simulink model "20240115_HVDCMMCInterconnection"  (R2023b)
settings: Solver=FixedStepDiscrete  StartTime=0.0  StopTime=2  FixedStep=Ts_Power  RelTol=1e-4  EnableMultiTasking=on
PreLoadFcn:
  | HVDCMMCInterconnectionParam
StartFcn:
  | tic
StopFcn:
  | toc
values from neighbouring files (symbols this model uses):
  C_PM = 1.758e-3    (= 0.001758)    [HVDCMMCInterconnectionParam.m]
  Cg = 50e-9    (= 5e-08)    [HVDCMMCInterconnectionParam.m]
  D_R = 0.001    [HVDCMMCInterconnectionParam.m]
  D_Rs = 1e8    (= 100000000)    [HVDCMMCInterconnectionParam.m]
  D_Vf = 0    [HVDCMMCInterconnectionParam.m]
  Fnom = 50    [HVDCMMCInterconnectionParam.m]
  HRM = 2    [HVDCMMCInterconnectionParam.m]
  Ki_Ireg = 6    [HVDCMMCInterconnectionParam.m]
  Ki_Preg = 1.0    (= 1)    [HVDCMMCInterconnectionParam.m]
  Ki_Qreg = 1.0    (= 1)    [HVDCMMCInterconnectionParam.m]
  Ki_VDCreg = 100    [HVDCMMCInterconnectionParam.m]
  Kp_Ireg = 0.6    [HVDCMMCInterconnectionParam.m]
  Kp_Preg = 0.5/3    (= 0.166666666667)    [HVDCMMCInterconnectionParam.m]
  Kp_Qreg = 0.5/3    (= 0.166666666667)    [HVDCMMCInterconnectionParam.m]
  Kp_VDCreg = 4    [HVDCMMCInterconnectionParam.m]
  L_cable = 15e-3    (= 0.015)    [HVDCMMCInterconnectionParam.m]
  Larm = Larm_pu*(Zb_ac/(2*pi*Fnom))    [HVDCMMCInterconnectionParam.m]
  Lff = Larm_pu/2    (= 0.075)    [HVDCMMCInterconnectionParam.m]
  Limits_Ireg = [ 2.0  -2.0]    [HVDCMMCInterconnectionParam.m]
  Limits_Preg = [ 1.2, 0.8 ]    [HVDCMMCInterconnectionParam.m]
  Limits_Qreg = [ 0.25, -0.25 ]    [HVDCMMCInterconnectionParam.m]
  Limits_VDCreg = [ 2.0  -2.0]    [HVDCMMCInterconnectionParam.m]
  Lxfo = 0.12    [HVDCMMCInterconnectionParam.m]
  Nb_PM = 36    [HVDCMMCInterconnectionParam.m]
  Pnom = 1000e6    (= 1000000000)    [HVDCMMCInterconnectionParam.m]
  R_cable = 0.5    [HVDCMMCInterconnectionParam.m]
  R_startup = 400    [HVDCMMCInterconnectionParam.m]
  Rarm = Rarm_pu*Zb_ac    [HVDCMMCInterconnectionParam.m]
  Rff = Rarm_pu/2    (= 0.00075)    [HVDCMMCInterconnectionParam.m]
  Rg = 100    [HVDCMMCInterconnectionParam.m]
  Rxfo = 0.003    [HVDCMMCInterconnectionParam.m]
  Slope_Pref = 0.5    [HVDCMMCInterconnectionParam.m]
  Slope_Qref = 0.5    [HVDCMMCInterconnectionParam.m]
  Slope_Vdc_ref = Vnom_dc/5    (= 128000)    [HVDCMMCInterconnectionParam.m]
  Tbrk1_On = 0.1    [HVDCMMCInterconnectionParam.m]
  Tbrk2_On = 1.0    (= 1)    [HVDCMMCInterconnectionParam.m]
  Tdeblock = 1.5    [HVDCMMCInterconnectionParam.m]
  Tfault = 9999    [HVDCMMCInterconnectionParam.m]
  Ton_Converter2 = 4    [HVDCMMCInterconnectionParam.m]
  Ton_PQreg = 4    [HVDCMMCInterconnectionParam.m]
  Ton_VDCreg = 1.5    [HVDCMMCInterconnectionParam.m]
  Ts = Ts_Control    (= 4e-05)    [HVDCMMCInterconnectionParam.m]
  Ts_Control = 40e-6    (= 4e-05)    [HVDCMMCInterconnectionParam.m]
  Ts_Power = 20e-6    (= 2e-05)    [HVDCMMCInterconnectionParam.m]
  Vb_ac = sqrt(2/3)*Vnom_sec    [HVDCMMCInterconnectionParam.m]
  Vb_dc = Vnom_dc    (= 640000)    [HVDCMMCInterconnectionParam.m]
  Vc0_PM = 0    [HVDCMMCInterconnectionParam.m]
  Vnom_dc = 640e3    (= 640000)    [HVDCMMCInterconnectionParam.m]
  Vnom_prim = 400e3    (= 400000)    [HVDCMMCInterconnectionParam.m]
  Vnom_sec = 333e3    (= 333000)    [HVDCMMCInterconnectionParam.m]
  w = 2*pi*Fnom    (= 314.159265359)    [HVDCMMCInterconnectionParam.m]
undefined symbols (not defined in the file or in its folder): ACDC3, DiscIntNeverNeededParam, gcbh, Pcc, sps_AC, sps_rtmsupport
libraries: simulink x38, spsControlledVoltageSourceLib x36, spsCurrentMeasurementLib x36, spsSeriesRLCBranchLib x26, spsDiodeLib x20, spsVoltageMeasurementLib x18, spsThreePhaseSeriesRLCBranchLib x7, spsGroundLib x7, spsHalfBridgeMMCmodel x4, powerlib_extras x3, spsMultimeterLib x3, spsThreePhaseBreakerLib x2
(part 1 of 7)
settings Model: Creator=The MathWorks, Inc.  LastModifiedBy=rober
settings SolverCC: ConcurrentTasks=on  ZeroCrossAlgorithm=Adaptive  InsertRTBMode=Always
settings DataIOCC: SaveFormat=StructureWithTime  SaveOutput=off  SignalLogging=off  DSMLogging=off  SaveTime=off  ReturnWorkspaceOutputs=off
settings OptimizationCC: ReuseModelBlockBuffer=off  ExpressionDepthLimit=2147483647  LifeSpan=inf
settings DebuggingCC: UnderspecifiedInitializationDetection=Classic  MergeDetectMultiDrivingBlocksExec=none  SolverPrmCheckMsg=warning  FcnCallInpInsideContextMsg=warning  AllowSymbolicDim=off  StateNameClashWarn=warning  SFUnexpectedBacktrackingDiag=warning  SFNoUnconditionalDefaultTransitionDiag=warning  SFExecutionAtInitializationDiag=none  ArithmeticOperatorsInVariantConditions=warning
settings HardwareCC: ProdBitPerPointer=32  ProdBitPerSizeT=32  ProdBitPerPtrDiffT=32  ProdLargestAtomicFloat=None  ProdIntDivRoundTo=Undefined  ProdEndianess=Unspecified  ProdWordSize=32  ProdHWDeviceType=32-bit Generic
settings ModelReferenceCC: EnableRefExpFcnMdlSchedulingChecks=on  EnableParallelModelReferenceBuilds=on  ModelReferenceMinAlgLoopOccurrences=on  PropagateSignalLabelsOutOfModel=off  UseModelRefSolver=on
settings SFSimCC: SimUseLocalCustomCode=off  CustomCodeUndefinedFunction=UseInterfaceOnly
settings RTWCC: RTWUseLocalCustomCode=off
settings CodeAppCC: StateflowObjectComments=on
settings GRTTargetCC: CombineOutputUpdateFcns=off  GRTInterface=on
settings ConfigComp: CovMetricSettings=dw  CovSaveCumulativeToWorkspaceVar=on  CovSaveSingleToWorkspaceVar=on  CovExternalEMLEnable=off
settings SimscapeCC: SimscapeNormalizeSystem=off

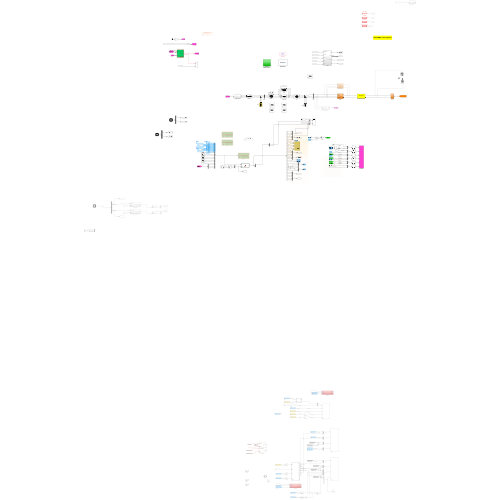
[thumbnail: Simulink's stored preview of the top-level diagram]
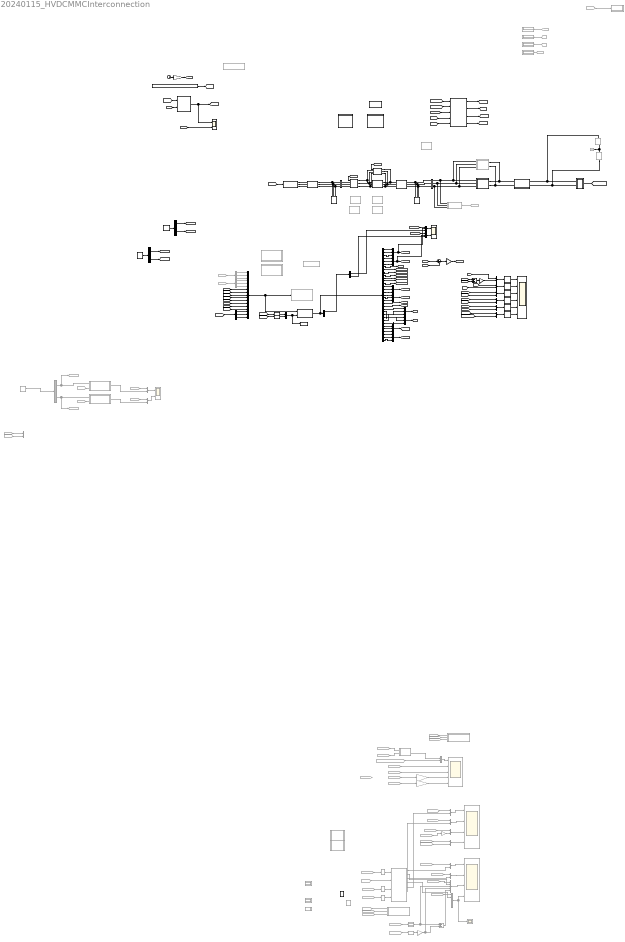
== system 20240115_HVDCMMCInterconnection ==
  note: HVDC-MMC Control System
  3ph SM1 : Subsystem  Commented=on
  3ph SM2 : Subsystem  Commented=on
  Add1 : Sum  Inputs=-+
  BRK_CTRL : Subsystem  Commented=on
  BRK_CTRL1 : Subsystem  Commented=on
  Brk1 : spsThreePhaseBreakerLib/Three-Phase Breaker  InitialState=open  SwitchA=on  SwitchB=on  SwitchC=on  SwitchTimes=0.1  External=on  BreakerResistance=0.01  SnubberResistance=1e6  SnubberCapacitance=inf  Measurements=Breaker voltages and currents
  Brk1_RS : spsThreePhaseSeriesRLCBranchLib/Three-Phase Series RLC Branch  Commented=on  LConnTagsString=A|B|C  RConnTagsString=A|B|C  BranchType=R  Resistance=1e6  Inductance=Vnom_prim^2 / Pcc / (2*pi*Fnom)  Capacitance=1e-6  Measurements=None
  Brk1_Ron : spsThreePhaseSeriesRLCBranchLib/Three-Phase Series RLC Branch  Commented=on  LConnTagsString=A|B|C  RConnTagsString=A|B|C  BranchType=R  Resistance=0.009  Inductance=Vnom_prim^2 / Pcc / (2*pi*Fnom)  Capacitance=1e-6  Measurements=None
  Brk2 : spsThreePhaseBreakerLib/Three-Phase Breaker  InitialState=open  SwitchA=on  SwitchB=on  SwitchC=on  SwitchTimes=[30/60]*10000  External=on  BreakerResistance=0.011  SnubberResistance=1e6  SnubberCapacitance=inf  Measurements=Breaker voltages and currents
  Brk2_RS : spsThreePhaseSeriesRLCBranchLib/Three-Phase Series RLC Branch  Commented=on  LConnTagsString=A|B|C  RConnTagsString=A|B|C  BranchType=R  Resistance=1e6  Inductance=Vnom_prim^2 / Pcc / (2*pi*Fnom)  Capacitance=1e-6  Measurements=None
  Brk2_Ron : spsThreePhaseSeriesRLCBranchLib/Three-Phase Series RLC Branch  Commented=on  LConnTagsString=A|B|C  RConnTagsString=A|B|C  BranchType=R  Resistance=0.011  Inductance=Vnom_prim^2 / Pcc / (2*pi*Fnom)  Capacitance=1e-6  Measurements=None
  COMPARE1 : Scope  NumInputPorts=6
  Cast To Double : DataTypeConversion  OutDataTypeStr=double  SaturateOnIntegerOverflow=off  RndMeth=Floor
  Cast To Double1 : DataTypeConversion  OutDataTypeStr=double  SaturateOnIntegerOverflow=off  RndMeth=Floor
  Clock : Clock
  Constant3 : Constant  Value=complex( [[ 0 Vnom_prim*sqrt(2/3); 0 0; 0 0] zeros(3,HRM-1) ])
  Control : Subsystem
  Conv 2 : Subsystem
      settings: PortSchema="{\"entries\":[{\"content\":{\"sides\":[{\"content\":{\"connectorIds\":[\"LConn1\",\"LConn2\"]},\"type\":\"ConnectorPlacement.EquallySpacedRectSide\",\"uuid\":\"34e68c3c-08e2-4036-96f4-bd6ca1a4adc7\"},{\"content\":{\"connectorIds\":[\"In1\"],\"side\":\"RIGHT\"},\"type\":\"ConnectorPlacement.EquallySpacedRectSide\",\"uuid\":\"8026f2da-b291-4e86-8efa-4dfa5391ad34\"},{\"content\":{\"side\":\"TOP\"},\"type\":\"ConnectorPlacement.EquallySpacedRectSide\",\"uuid\":\"2a5049d1-3deb-4ece-8237-adb3b31cd77f\"}]},\"type\":\"ConnectorPlacement.EquallySpacedConnector\",\"uuid\":\"95075630-e580-4539-9cf3-c9c75bab0a7f\"}],\"packageUris\":[\"http://schema.mathworks.com/mf0/Connector/R2020b\"],\"version\":\"1.0\"}"
  DC & converter 2 : Subsystem
      mask Display: disp('DC circuit')
  DQn->ABC : MATLAB Function  TreatAsAtomicUnit=on  SystemSampleTime=Ts_Power  mask{N=HRM}
      mask prompts: N "Harmonic order:"
  DSS : Subsystem  Commented=on  SystemSampleTime=Ts_Power  mask{A=ACDC3.A, B=ACDC3.B, C=ACDC3.C, D=ACDC3.D, InitVec=ACDC3.x0, dt=Ts_Power, DQSYM=off, N=HRM, Ws=w}
      mask prompts: InitVec "Initial condition:"; dt "Time step (s):"; N "Harmonic number:"; Ws "Angular frequency (1/rad):"
      mask init:
      | % I = eye(size(A,1));
      | % INVR = I/(I-A*dt/2);
      | % Ad1 = INVR*(I+A*dt/2);
      | % Bd1 = INVR*B*dt/2;
      | % Cd1 = C*Ad1;
      | % Dd11 = C*INVR*B*dt/2+D;
      | % Dd12 = C*INVR*B*dt/2;
      | 
      |     I = eye(size(A,1));
      |     INVR = I/(I-A*dt/2);
      |     Ad1 = INVR*(I+A*dt/2);
      |     Bd1 = INVR*B;
      |     Cd1 = C*INVR*dt;
      |     Dd1 = Cd1*B/2 + D;
      | 
      | DQSYM = get_param(gcb,'DQSYM');
      | 
      | comp = 0;
      | 
      | if(strcmp(DQSYM,'on'))
      | 
      | %Calculating the PNZ matrices
      | 
      |     a = -0.5+0.866i;
      |     a2 = -0.5-0.866i;
      |     Sas = [1,a,a2;1,a2,a;1,1,1]/3;
      | 
      |     arows = size(Ad1,1)/3; %signal size
      |     acols = size(Ad1,2)/3; %signal size
      | 
      |     brows = size(Bd1,1)/3; %signal size
      |     bcols = size(Bd1,2)/3; %signal size
      | 
      |     crows = size(Cd1,1)/3; %signal size
      |     ccols = size(Cd1,2)/3; %signal size
      | 
      |     d1rows = size(Dd1,1)/3; %signal size
      |     d1cols = size(Dd1,2)/3; %signal size
      | 
      |     %%%%%%%%%%%%%%%%%%%%%%% Check for inconsistencies  %%%%%%%%%%%%%%%%%%%%%%%
      | 
      |     szMatA = size(A,1);
      |     iL = eye(szMatA);
      |     szMatiL = size(iL,1);
      | 
      |     if(szMatiL ~= szMatA || size(A,1) ~= size(A,2) || size(iL,1) ~= size(iL,2))
      |         error('[Int_DQN_Mat/swFeedback] check matrix A size!');
      |     end
      | 
      |     if(arows ~= brows || acols ~= ccols || crows ~= d1rows || bcols ~= d1cols)
      |         error('[Int_DQN_Mat/Initialize] the sizes of the state-space matrices!');
      |     end
      | 
      |     %%%%%%%%%%%%%%%%%%%%%%%%%%%%%%%%%%%%%%%%%%%%%%%%%%%%%%%%%%%%%%%
      | 
      | 
      |     %%%%%%%%%%%%%%%%%%%%%%% A --> Bpnz %%%%%%%%%%%%%%%%%%%%%%%
      |     Adc = complex(zeros(3*arows,3*acols));
      | 
      |     for i = 1 : arows
      |         for j = 1 : acols
      |             Adc((1:3) + (i-1)*3,(1:3) + (j-1)*3) = Sas*Ad1((1:3) + (i-1)*3,(1:3) + (j-1)*3)/Sas;
      |             %Adc((1:3) + (i-1)*3,(1:3) + (j-1)*3) = diag(diag(real(Adc((1:3) + (i-1)*3,(1:3) + (j-1)*3))));
      |             %Adc((1:3) + (i-1)*3,(1:3) + (j-1)*3) = diag(diag((Adc((1:3) + (i-1)*3,(1:3) + (j-1)*3))));
      | 
      |         end
      |     end
      |     %%%%%%%%%%%%%%%%%%%%%%%%%%%%%%%%%%%%%%%%%%%%%%%%%%%%%%%%%%%%%%%
      | 
      |     %%%%%%%%%%%%%%%%%%%%%%% B --> Bpnz %%%%%%%%%%%%%%%%%%%%%%%
      | 
      |     Bdc = complex(zeros(3*brows,3*bcols));
      | 
      |     for i = 1 : brows
      |         for j = 1 : bcols
      |             Bdc((1:3) + (i-1)*3,(1:3) + (j-1)*3) = Sas*Bd1((1:3) + (i-1)*3,(1:3) + (j-1)*3)/Sas;
      |             %Bdc((1:3) + (i-1)*3,(1:3) + (j-1)*3) = diag(diag(real(Bdc((1:3) + (i-1)*3,(1:3) + (j-1)*3))));
      |             %Bdc((1:3) + (i-1)*3,(1:3) + (j-1)*3) = diag(diag((Bdc((1:3) + (i-1)*3,(1:3) + (j-1)*3))));
      | 
      |         end
      |     end
      |     %%%%%%%%%%%%%%%%%%%%%%%%%%%%%%%%%%%%%%%%%%%%%%%%%%%%%%%%%%%%%%%
      | 
      |     %%%%%%%%%%%%%%%%%%%%%%% C --> Cpnz %%%%%%%%%%%%%%%%%%%%%%%
      | 
      |     Cdc = complex(zeros(3*crows,3*ccols));
      | 
      |     for i = 1 : crows
      |         for j = 1 : ccols
      |             Cdc((1:3) + (i-1)*3,(1:3) + (j-1)*3) = Sas*Cd1((1:3) + (i-1)*3,(1:3) + (j-1)*3)/Sas;
      |             %Cdc((1:3) + (i-1)*3,(1:3) + (j-1)*3) = diag(diag(real(Cdc((1:3) + (i-1)*3,(1:3) + (j-1)*3))));
      |             %Cdc((1:3) + (i-1)*3,(1:3) + (j-1)*3) = diag(diag((Cdc((1:3) + (i-1)*3,(1:3) + (j-1)*3))));
      |         end
      |     end
      |     %%%%%%%%%%%%%%%%%%%%%%%%%%%%%%%%%%%%%%%%%%%%%%%%%%%%%%%%%%%%%%%
      | 
      |     
      |     %%%%%%%%%%%%%%%%%%%%%%% D1 --> Cpnz %%%%%%%%%%%%%%%%%%%%%%%
      | 
      |     Ddc = complex(zeros(3*d1rows,3*d1cols));
      | 
      |     for i = 1 : d1rows
      |         for j = 1 : d1cols
      |             Ddc((1:3) + (i-1)*3,(1:3) + (j-1)*3) = Sas*Dd1((1:3) + (i-1)*3,(1:3) + (j-1)*3)/Sas;
      |             %Ddc1((1:3) + (i-1)*3,(1:3) + (j-1)*3) = diag(diag(real(Ddc1((1:3) + (i-1)*3,(1:3) + (j-1)*3))));
      |             %Ddc((1:3) + (i-1)*3,(1:3) + (j-1)*3) = diag(diag((Ddc((1:3) + (i-1)*3,(1:3) + (j-1)*3))));
      |         end
      |     end
      |     %%%%%%%%%%%%%%%%%%%%%%%%%%%%%%%%%%%%%%%%%%%%%%%%%%%%%%%%%%%%%%%
      | 
      |     Adc(abs(Adc)<2*eps) = 0;
      |     Bdc(abs(Bdc)<2*eps) = 0;
      |     Cdc(abs(Cdc)<2*eps) = 0;
      |     Ddc(abs(Ddc)<2*eps) = 0;
      | 
      |     InitVec_c = complex(zeros(brows*3,N+1));
      | 
      | 
      |     if(~isempty(InitVec))
      |         if(mod(numel(InitVec),3)~=0) 
      |             warning('[SS_DQNc_Mat] InitVec with wrong size --> needs to be a multiple of 3!'); 
      | 
      |         else
      |             for k = 1 : numel(InitVec)/3
      |                 InitVec_c((k-1)*3+1:(k-1)*3+3,1) = Sas*InitVec((k-1)*3+1:(k-1)*3+3)*exp(+1i*Ws*dt);
      |             end
      |         end
      |     end
      | 
      |     InitVec = InitVec_c;
      | 
      | 
      |     Ad1 = Adc;
      |     Bd1 = Bdc;
      |     Cd1 = Cdc;
      |     Dd1 = Ddc;
      | 
      |     comp = -1i*Ws*dt;
      | 
      | end
      settings: MinAlgLoopOccurrences=on
      settings: LibrarySourceBlock=|
      | spsSynchronousMachineModel/Discrete robust/State Space Model/Discretize
      | BE or Tustin
      mask Callback DQSYM:
      | EMT = get_param(gcb,'DQSYM');
      | 
      | if(strcmp(EMT,'on'))
      |    set_param(gcb,'MaskVisibilities',{'on','on','on','on','on','on','on','on','on'});
      | else
      |    set_param(gcb,'MaskVisibilities',{'on','on','on','on','on','on','on','off','off'});
      | end
      mask Display: disp(['{\color{red}\bf\fontsize{12}x(t) = Ad*x(t-dt)+Bd*u(t)}',newline,'{\color{gray}\bf\fontsize{12}y(t) = Cd*x(t-dt)+Dd*u(t)}'], 'texmode','on');
  DSS1 : Subsystem  Commented=on  SystemSampleTime=Ts_Power  mask{A=ACDC3.A, B=ACDC3.B, C=ACDC3.C, D=ACDC3.D, InitVec=ACDC3.x0, dt=Ts_Power, NrBrk=6, DQSYM=off, N=HRM, Ws=w}
      mask prompts: InitVec "Initial condition:"; dt "Time step (s):"; NrBrk "Number of breakers:"; N "Harmonic number:"; Ws "Angular frequency (1/rad):"
      mask init:
      | % I = eye(size(A,1));
      | % INVR = I/(I-A*dt/2);
      | % Ad1 = INVR*(I+A*dt/2);
      | % Bd1 = INVR*B*dt/2;
      | % Cd1 = C*Ad1;
      | % Dd11 = C*INVR*B*dt/2+D;
      | % Dd12 = C*INVR*B*dt/2;
      | 
      |     I = eye(size(A,1));
      |     INVR = I/(I-A*dt/2);
      |     Ad1 = INVR*(I+A*dt/2);
      |     Bd1 = INVR*B;
      |     Cd1 = C*INVR*dt;
      |     Dd1 = Cd1*B/2 + D;
      | 
      | DQSYM = get_param(gcb,'DQSYM');
      | 
      | comp = 0;
      | 
      |     arows = size(Ad1,1)/3; %signal size
      |     acols = size(Ad1,2)/3; %signal size
      | 
      |     brows = size(Bd1,1)/3; %signal size
      |     bcols = size(Bd1,2)/3; %signal size
      | 
      |     crows = size(Cd1,1)/3; %signal size
      |     ccols = size(Cd1,2)/3; %signal size
      | 
      |     d1rows = size(Dd1,1)/3; %signal size
      |     d1cols = size(Dd1,2)/3; %signal size
      | 
      | if(strcmp(DQSYM,'on'))
      | 
      | %Calculating the PNZ matrices
      | 
      |     a = -0.5+0.866i;
      |     a2 = -0.5-0.866i;
      |     Sas = [1,a,a2;1,a2,a;1,1,1]/3;
      | 
      | 
      | 
      |     %%%%%%%%%%%%%%%%%%%%%%% Check for inconsistencies  %%%%%%%%%%%%%%%%%%%%%%%
      | 
      |     szMatA = size(A,1);
      |     iL = eye(szMatA);
      |     szMatiL = size(iL,1);
      | 
      |     if(szMatiL ~= szMatA || size(A,1) ~= size(A,2) || size(iL,1) ~= size(iL,2))
      |         error('[Int_DQN_Mat/swFeedback] check matrix A size!');
      |     end
      | 
      |     if(arows ~= brows || acols ~= ccols || crows ~= d1rows || bcols ~= d1cols)
      |         error('[Int_DQN_Mat/Initialize] the sizes of the state-space matrices!');
      |     end
      | 
      |     %%%%%%%%%%%%%%%%%%%%%%%%%%%%%%%%%%%%%%%%%%%%%%%%%%%%%%%%%%%%%%%
      | 
      | 
      |     %%%%%%%%%%%%%%%%%%%%%%% A --> Bpnz %%%%%%%%%%%%%%%%%%%%%%%
      |     Adc = complex(zeros(3*arows,3*acols));
      | 
      |     for i = 1 : arows
      |         for j = 1 : acols
      |             Adc((1:3) + (i-1)*3,(1:3) + (j-1)*3) = Sas*Ad1((1:3) + (i-1)*3,(1:3) + (j-1)*3)/Sas;
      |             %Adc((1:3) + (i-1)*3,(1:3) + (j-1)*3) = diag(diag(real(Adc((1:3) + (i-1)*3,(1:3) + (j-1)*3))));
      |             %Adc((1:3) + (i-1)*3,(1:3) + (j-1)*3) = diag(diag((Adc((1:3) + (i-1)*3,(1:3) + (j-1)*3))));
      | 
      |         end
      |     end
      |     %%%%%%%%%%%%%%%%%%%%%%%%%%%%%%%%%%%%%%%%%%%%%%%%%%%%%%%%%%%%%%%
      | 
      |     %%%%%%%%%%%%%%%%%%%%%%% B --> Bpnz %%%%%%%%%%%%%%%%%%%%%%%
      | 
      |     Bdc = complex(zeros(3*brows,3*bcols));
      | 
      |     for i = 1 : brows
      |         for j = 1 : bcols
      |             Bdc((1:3) + (i-1)*3,(1:3) + (j-1)*3) = Sas*Bd1((1:3) + (i-1)*3,(1:3) + (j-1)*3)/Sas;
      |             %Bdc((1:3) + (i-1)*3,(1:3) + (j-1)*3) = diag(diag(real(Bdc((1:3) + (i-1)*3,(1:3) + (j-1)*3))));
      |             %Bdc((1:3) + (i-1)*3,(1:3) + (j-1)*3) = diag(diag((Bdc((1:3) + (i-1)*3,(1:3) + (j-1)*3))));
      | 
      |         end
      |     end
      |     %%%%%%%%%%%%%%%%%%%%%%%%%%%%%%%%%%%%%%%%%%%%%%%%%%%%%%%%%%%%%%%
      | 
      |     %%%%%%%%%%%%%%%%%%%%%%% C --> Cpnz %%%%%%%%%%%%%%%%%%%%%%%
      | 
      |     Cdc = complex(zeros(3*crows,3*ccols));
      | 
      |     for i = 1 : crows
      |         for j = 1 : ccols
      |             Cdc((1:3) + (i-1)*3,(1:3) + (j-1)*3) = Sas*Cd1((1:3) + (i-1)*3,(1:3) + (j-1)*3)/Sas;
      |             %Cdc((1:3) + (i-1)*3,(1:3) + (j-1)*3) = diag(diag(real(Cdc((1:3) + (i-1)*3,(1:3) + (j-1)*3))));
      |             %Cdc((1:3) + (i-1)*3,(1:3) + (j-1)*3) = diag(diag((Cdc((1:3) + (i-1)*3,(1:3) + (j-1)*3))));
      |         end
      |     end
      |     %%%%%%%%%%%%%%%%%%%%%%%%%%%%%%%%%%%%%%%%%%%%%%%%%%%%%%%%%%%%%%%
      | 
      |     
      |     %%%%%%%%%%%%%%%%%%%%%%% D1 --> Cpnz %%%%%%%%%%%%%%%%%%%%%%%
      | 
      |     Ddc = complex(zeros(3*d1rows,3*d1cols));
      | 
      |     for i = 1 : d1rows
      |         for j = 1 : d1cols
      |             Ddc((1:3) + (i-1)*3,(1:3) + (j-1)*3) = Sas*Dd1((1:3) + (i-1)*3,(1:3) + (j-1)*3)/Sas;
      |             %Ddc1((1:3) + (i-1)*3,(1:3) + (j-1)*3) = diag(diag(real(Ddc1((1:3) + (i-1)*3,(1:3) + (j-1)*3))));
      |             %Ddc((1:3) + (i-1)*3,(1:3) + (j-1)*3) = diag(diag((Ddc((1:3) + (i-1)*3,(1:3) + (j-1)*3))));
      |         end
      |     end
      |     %%%%%%%%%%%%%%%%%%%%%%%%%%%%%%%%%%%%%%%%%%%%%%%%%%%%%%%%%%%%%%%
      | 
      |     Adc(abs(Adc)<2*eps) = 0;
      |     Bdc(abs(Bdc)<2*eps) = 0;
      |     Cdc(abs(Cdc)<2*eps) = 0;
      |     Ddc(abs(Ddc)<2*eps) = 0;
      | 
      |     InitVec_c = complex(zeros(brows*3,N+1));
      | 
      | 
      |     if(~isempty(InitVec))
      |         if(mod(numel(InitVec),3)~=0) 
      |             warning('[SS_DQNc_Mat] InitVec with wrong size --> needs to be a multiple of 3!'); 
      | 
      |         else
      |             for k = 1 : numel(InitVec)/3
      |                 InitVec_c((k-1)*3+1:(k-1)*3+3,1) = Sas*InitVec((k-1)*3+1:(k-1)*3+3)*exp(+1i*Ws*dt);
      |             end
      |         end
      |     end
      | 
      |     InitVec = InitVec_c;
      | 
      | 
      |     Ad1 = Adc;
      |     Bd1 = Bdc;
      |     Cd1 = Cdc;
      |     Dd1 = Ddc;
      | 
      |     comp = -1i*Ws*dt;
      | 
      | 
      | end
      | 
      |     
      |     Ad11 = Ad1(1:NrBrk,1:NrBrk);        if(isempty(Ad11)) Ad11 = zeros(3,3); end
      |     Ad12 = Ad1(1:NrBrk,NrBrk+1:end);    if(isempty(Ad12)) Ad12 = zeros(3,3); end
      |     Ad21 = Ad1(NrBrk+1:end,1:NrBrk);    if(isempty(Ad21)) Ad21 = zeros(3,3); end
      |     Ad22 = Ad1(NrBrk+1:end,NrBrk+1:end); if(isempty(Ad22)) Ad22 = zeros(3,3); end
      | 
      |     Bd11 = Bd1(1:NrBrk,1:NrBrk);        if(isempty(Bd11)) Bd11 = zeros(3,3); end
      |     Bd12 = Bd1(1:NrBrk,NrBrk+1:end);    if(isempty(Bd12)) Bd12 = zeros(3,3); end
      |     Bd21 = Bd1(NrBrk+1:end,1:NrBrk);    if(isempty(Bd21)) Bd21 = zeros(3,3); end
      |     Bd22 = Bd1(NrBrk+1:end,NrBrk+1:end); if(isempty(Bd22)) Bd22 = zeros(3,3*bcols-NrBrk); end
      | 
      |     Cd11 = Cd1(1:NrBrk,1:NrBrk);        if(isempty(Cd11)) Cd11 = zeros(3,3); end
      |     Cd12 = Cd1(1:NrBrk,NrBrk+1:end);    if(isempty(Cd12)) Cd12 = zeros(3,3); end
      |     Cd21 = Cd1(NrBrk+1:end,1:NrBrk);    if(isempty(Cd21)) Cd21 = zeros(3,3); end
      |     Cd22 = Cd1(NrBrk+1:end,NrBrk+1:end); if(isempty(Cd22)) Cd22 = zeros(3*crows-NrBrk,3*ccols); end
      | 
      |     Dd11 = Dd1(1:NrBrk,1:NrBrk);        if(isempty(Dd11)) Dd11 = zeros(3,3); end
      |     Dd12 = Dd1(1:NrBrk,NrBrk+1:end);    if(isempty(Dd12)) Dd12 = zeros(3,3); end
      |     Dd21 = Dd1(NrBrk+1:end,1:NrBrk);    if(isempty(Dd21)) Dd21 = zeros(3,3); end
      |     Dd22 = Dd1(NrBrk+1:end,NrBrk+1:end); if(isempty(Dd22)) Dd22 = zeros(3,3); end
      | 
      | 
      | 
      | 
      | InitVecS = InitVec(1:NrBrk);
      | 
      | InitVecNS = InitVec(NrBrk+1:end); if(isempty(InitVecNS)) InitVecNS = 0; end
      settings: MinAlgLoopOccurrences=on
      settings: LibrarySourceBlock=|
      | spsSynchronousMachineModel/Discrete robust/State Space Model/Discretize
      | BE or Tustin
      mask Display: disp(['{\color{red}\bf\fontsize{12}x(t) = Ad*x(t-dt)+Bd*u(t)}',newline,'{\color{gray}\bf\fontsize{12}y(t) = Cd*x(t-dt)+Dd*u(t)}'], 'texmode','on');
  DSS2 : Subsystem  Commented=on  SystemSampleTime=Ts_Power  mask{A=ACDC3.A, B=ACDC3.B, C=ACDC3.C, D=ACDC3.D, InitVec=ACDC3.x0, dt=Ts_Power, NrBrk=6, DQSYM=off, N=HRM, Ws=w}
      mask prompts: InitVec "Initial condition:"; dt "Time step (s):"; NrBrk "Number of breakers:"; N "Harmonic number:"; Ws "Angular frequency (1/rad):"
      mask init: same as 20240115_HVDCMMCInterconnection/DSS1
      settings: MinAlgLoopOccurrences=on
      settings: LibrarySourceBlock=|
      | spsSynchronousMachineModel/Discrete robust/State Space Model/Discretize
      | BE or Tustin
      mask Display: disp(['{\color{red}\bf\fontsize{12}x(t) = Ad*x(t-dt)+Bd*u(t)}',newline,'{\color{gray}\bf\fontsize{12}y(t) = Cd*x(t-dt)+Dd*u(t)}'], 'texmode','on');
  Delay{,3,10..11} (4 alike) : Delay  Commented=on  DelayLength=1  SampleTime=Ts_Power
  Delay2 : Delay  DelayLength=1  SampleTime=Ts_Power
  Delay5 : Subsystem  Commented=on
  Delay6 : Subsystem  Commented=on
  Delay7 : Subsystem  Commented=on
  Delay8 : Subsystem  Commented=on
  Delay9 : Subsystem  Commented=on
  Demux : Demux  Outputs=2
  Demux1 : Demux  Commented=on  Outputs=3
  Demux2 : Demux  Commented=on  Outputs=3
  Demux3 : Demux  Outputs=3
  Demux4 : Demux  Commented=on  Outputs=2
  Demux5 : Demux  Outputs=2
  Demux6 : Demux  Outputs=numel(ACDC3.outputs)
  Demux7 : Demux  Outputs=[6,27]
  Demux8 : Demux  Outputs=2
  Discrete State-Space : DiscreteStateSpace  Commented=on  A=ACDC3.Adiscrete  B=ACDC3.Bdiscrete  C=ACDC3.Cdiscrete  D=ACDC3.Ddiscrete  InitialCondition=ACDC3.x0  SampleTime=Ts_Power
  From : From  Commented=on  GotoTag=Uref_Ap  TagVisibility=global
  From1 : From  Commented=on  GotoTag=Uref_An  TagVisibility=global
  From10 : From  Commented=on  GotoTag=IBrk2_EMT  TagVisibility=global
  From102 : From  Commented=on  GotoTag=Ap_Vin  TagVisibility=global
  From103 : From  Commented=on  GotoTag=Ap_Vbl  TagVisibility=global
  From107 : From  Commented=on  GotoTag=I_Ap_Db  TagVisibility=global
  From11 : From  Commented=on  GotoTag=Q
  From{27,44,48,113} (4 alike) : From  Commented=on  GotoTag=I_Ap_Dt  TagVisibility=global
  From118 : From  Commented=on  GotoTag=I_Ap_Db  TagVisibility=global
  From119 : From  Commented=on  GotoTag=Ap_Icap
  From{36..37,91,120} (4 alike) : From  Commented=on  GotoTag=Ap_Ipos
  From2 : From  Commented=on  GotoTag=P
  From25 : From  Commented=on  GotoTag=Brk1_On  TagVisibility=global
  From26 : From  Commented=on  GotoTag=UBrk1_ss
  From28 : From  Commented=on  GotoTag=U_Ap_Dt
  From29 : From  Commented=on  GotoTag=Brk2_On  TagVisibility=global
  From30 : From  Commented=on  GotoTag=IBrk2_EMT  TagVisibility=global
  From31 : From  Commented=on  GotoTag=IBrk1_EMT  TagVisibility=global
  From33 : From  Commented=on  GotoTag=UBrk2_ss
  From34 : From  Commented=on  GotoTag=Uref_Ap  TagVisibility=global
  From39 : From  Commented=on  GotoTag=U_Ap_Dt
  From4 : From  Commented=on  GotoTag=Vdc_kV
  From5 : From  Commented=on  GotoTag=V1rmsLL
  From6 : From  Commented=on  GotoTag=Vsec_ABC
  From69 : From  Commented=on  GotoTag=U_Ap_SM
  From7 : From  Commented=on  GotoTag=An_Ipos
  From8 : From  Commented=on  GotoTag=IBrk1_EMT  TagVisibility=global
  From85 : From  Commented=on  GotoTag=Ap_Icap
  From9 : From  Commented=on  GotoTag=An_Icap
  From90 : From  Commented=on  GotoTag=Ap_Icap
  From96 : From  Commented=on  GotoTag=Uref_Ap  TagVisibility=global
  Gain1 : Gain  Commented=on  Gain=-1
  Gain2 : Gain  Commented=on  Gain=D_Rs/(D_R+D_Rs)
  Gain4 : Gain  Commented=on  Gain=1/Vb_dc
  Gain5 : Gain  Gain=2*pi*50
  Gain6 : Gain  Gain=0.5
  Gain7 : Gain  Commented=on  Gain=1/Vb_dc
  Goto12 : Goto  Commented=on  GotoTag=UBrk2_EMT  TagVisibility=global
  Goto13 : Goto  Commented=on  GotoTag=UBrk1_EMT  TagVisibility=global
  Ground2 : spsGroundLib/Ground  Commented=on  LConnTagsString=a
  I->pu1 : Gain  Gain=0.5  SaturateOnIntegerOverflow=on  OutDataTypeStr=Inherit: Same as input  ParamDataTypeStr=Inherit: Same as input
  Ld1 : spsThreePhaseSeriesRLCLoadLib/Three-Phase Series RLC Load  LConnTagsString=A|B|C  Configuration=Y (grounded)  NominalVoltage=Vnom_prim  Vabc=[1e3 1e3 1e3]  Vabcp=[1e3 1e3 1e3]  NominalFrequency=Fnom  UnbalancedPower=off  ActivePower=P_Ld1  InductivePower=0  CapacitivePower=0  Pabc=[10e3 9e3 11e3]  QLabc=[100 90 110]  QCabc=[100 90 110]  Pabcp=[10e3 9e3 11e3]  QLabcp=[100 90 110]  QCabcp=[100 90 110]  Measurements=None  LoadType=constant Z
  Ld2 : spsThreePhaseSeriesRLCLoadLib/Three-Phase Series RLC Load  LConnTagsString=A|B|C  Configuration=Y (grounded)  NominalVoltage=Vnom_sec  Vabc=[1e3 1e3 1e3]  Vabcp=[1e3 1e3 1e3]  NominalFrequency=Fnom  UnbalancedPower=off  ActivePower=500e3  InductivePower=0  CapacitivePower=0  Pabc=[10e3 9e3 11e3]  QLabc=[100 90 110]  QCabc=[100 90 110]  Pabcp=[10e3 9e3 11e3]  QLabcp=[100 90 110]  QCabcp=[100 90 110]  Measurements=None  LoadType=constant Z
  MATLAB Function : MATLAB Function  Commented=on  TreatAsAtomicUnit=on
  MATLAB Function1 : MATLAB Function  TreatAsAtomicUnit=on  mask{Ad=ACDC3.Adiscrete, Bd=ACDC3.Bdiscrete, Cd=ACDC3.Cdiscrete, Dd=ACDC3.Ddiscrete, InitVec=ACDC3.x0, dt=Ts_Power, nsw=6}
      mask prompts: Ad "A"; Bd "B"; Cd "C"; Dd "D"; InitVec "Initial values:"; dt "Time step (s):"; nsw "Number of switches:"
  MATLAB Function2 : MATLAB Function  Commented=on  SystemSampleTime=Ts_Power  mask{Ts=Ts_Power, D_R=D_R, D_Rs=D_Rs, Nb_SM=Nb_PM, C=C_PM}
      mask prompts: Ts "Time step (s):"; D_R "Resistance Ron (Ohms):"; D_Rs "Snubber resistance Rs (Ohms):"; Nb_SM "Number of submodules:"; C "Submodule capacitance (F):"
      settings: MinAlgLoopOccurrences=on
  MMC : Subsystem
  MMC_SS : Subsystem  Commented=on
  Model1 : Subsystem  Commented=on  AncestorBlock=spsDiodeModel/Discrete  mask(DiscreteModel){}
  Model2 : Subsystem  Commented=on  AncestorBlock=spsDiodeModel/Discrete  mask(DiscreteModel){}
  Multimeter : spsMultimeterLib/Multimeter  L=12  sel=[7 8 9 10 11 12]  yselected={}  Gain=[1 1 1 1 1 1]  OutputType=Complex  PlotAtSimulationStop=off  PhasorSimulation=off
  Multimeter1 : spsMultimeterLib/Multimeter  Commented=on  L=12  sel=[1 2 3 4 5 6]  yselected={}  Gain=[1 1 1 1 1 1]  OutputType=Complex  PlotAtSimulationStop=off  PhasorSimulation=off
  Multimeter2 : spsMultimeterLib/Multimeter  L=12  sel=[1 2 3 4 5 6]  yselected={}  Gain=[1 1 1 1 1 1]  OutputType=Complex  PlotAtSimulationStop=off  PhasorSimulation=off
  Mux{,1..7,12,14} (10 alike) : Mux  Inputs=3
  Mux{8..10,13,24,28,32..35} (10 alike) : Mux  Commented=on  Inputs=2
  Mux{11,38..43} (7 alike) : Mux  Inputs=2
  Mux23 : Mux  Inputs=numel(ACDC3.inputs)
  Mux29 : Mux  Commented=on  Inputs=5
  Mux30 : Mux  Commented=on  Inputs=5
  P (MW) : Display  Commented=on
      settings: Format=bank  Decimation=5000
  Q (Mvar) : Display  Commented=on
      settings: Format=bank  Decimation=5000
  RL Src : spsThreePhaseSeriesRLCBranchLib/Three-Phase Series RLC Branch  LConnTagsString=A|B|C  RConnTagsString=A|B|C  BranchType=RL  Resistance=0.8929  Inductance=16.58e-3  Capacitance=1e-6  Measurements=None
  R_startup : spsThreePhaseSeriesRLCBranchLib/Three-Phase Series RLC Branch  LConnTagsString=A|B|C  RConnTagsString=A|B|C  BranchType=R  Resistance=R_startup  Inductance=Vnom_prim^2 / Pcc / (2*pi*Fnom)  Capacitance=1e-6  Measurements=None
  R_startup2 : spsThreePhaseSeriesRLCBranchLib/Three-Phase Series RLC Branch  Commented=on  LConnTagsString=A|B|C  RConnTagsString=A|B|C  BranchType=R  Resistance=0.011  Inductance=Vnom_prim^2 / Pcc / (2*pi*Fnom)  Capacitance=1e-6  Measurements=None
  Rate Transition{,1..5} (6 alike) : RateTransition
  Scope : Scope  Commented=on  NumInputPorts=2
  Scope1 : Scope  NumInputPorts=2
  Scope2 : Scope  Commented=on  NumInputPorts=5
  Scope3 : Scope  Commented=on  NumInputPorts=4
  Scope5 : Scope  Commented=on  NumInputPorts=4
  Scope7 : Scope  Commented=on
  Scope8 : Scope  NumInputPorts=2
  Scopes & Measurements : Subsystem
  Sequencer : Subsystem
      mask Display: disp('Sequencer')
  Status : From  Commented=on  GotoTag=T43_3835_2986319703090  TagVisibility=global
      settings: CloseFcn=tagdialog Close
  Status_Bottom : From  Commented=on  GotoTag=T42_3768_2839018950081  TagVisibility=global
      settings: CloseFcn=tagdialog Close
  Status_Top : From  Commented=on  GotoTag=T43_3835_2986319703090  TagVisibility=global
      settings: CloseFcn=tagdialog Close
  Subtract : Sum  Commented=on  Inputs=+-
  Sum2 : Sum  Inputs=|+-
  To Workspace1 : ToWorkspace  VariableName=bvecsim  SampleTime=Ts_Power
      settings: Save2DSignal=2-D array (concatenate along first dimension)
  Tr1 : spsThreePhaseTransformerTwoWindingsLib/Three-Phase Transformer (Two Windings)  Winding1Connection=Yg  Winding2Connection=Yg  CoreType=Three single-phase transformers  SetSaturation=off  Hysteresis=off  DataFile='hysteresis'  SetInitialFlux=off  Measurements=None  UNITS=pu  NominalPower=[ Pnom , Fnom ]  Winding1="[ Vnom_prim , Rxfo/2,  Lxfo/2 ]"  Winding2="[ Vnom_sec , Rxfo/2,  Lxfo/2 ]"  Rm=1000  Lm=1000  L0=0.5  Saturation=[ 0,0 ; 0.0024,1.2 ; 1.0,1.52 ]  InitialFluxes=[ 0.8 , -0.8 , 0.7 ]  BreakLoop=off  DiscreteSolver=Trapezoidal iterative  DataType=off  TransfoNumber=1
  USW_Bottom : From  Commented=on  GotoTag=T43_3867_2942891286788  TagVisibility=global
  USW_Bottom1 : From  Commented=on  GotoTag=T43_3867_2942891286788  TagVisibility=global
  USW_Top2 : From  Commented=on  GotoTag=T44_3934_3096165412659  TagVisibility=global
  USW_Top3 : From  Commented=on  GotoTag=T44_3934_3096165412659  TagVisibility=global
  Uref2m1 : Subsystem  Commented=on
  V1 (kV rms LL) : Display  Commented=on
      settings: Format=bank  Decimation=5000
  VS Conv2b : spsControlledVoltageSourceLib/Controlled Voltage Source  Commented=on  Initialize=on  Source_Type=AC  Amplitude=0  Phase=0  Frequency=0  Measurements=None
  VS Conv2t : spsControlledVoltageSourceLib/Controlled Voltage Source  Commented=on  Initialize=on  Source_Type=AC  Amplitude=0  Phase=0  Frequency=0  Measurements=None
  Vdc (kV) : Display  Commented=on
      settings: Format=bank  Decimation=5000
  Voltage source : Subsystem
  Voltage source1 : Subsystem  Commented=on
  param : Subsystem  Commented=on
      settings: OpenFcn=open('HVDCMMCInterconnectionParam')
      mask Display: disp('Double-click to open\nparameters file')
  powergui : spspowerguiLib/powergui  Priority=1  SimulationMode=Discrete  SampleTime=Ts_Power  frequency=60  Iterations=50  frequencyindice=0  Pbase=100e6  ErrMax=1e-4  UnitsV=kV  UnitsW=MW  buscounter=0  FunctionMessages=off  echomessages=off  EnableUseOfTLC=off  CurrentSourceSwitches=off  DisableSnubberDevices=off  DisableRonSwitches=off  DisableVfSwitches=off  DisplayEquations=off  AutomaticDiscreteSolvers=off  SolverType=Tustin/Backward Euler (TBE)  Interpol=off  ExternalGateDelay=off  methode=off  Ts=10  x0status=blocks  SPID=off  SwTol=0  HookPort=off  NonlinearTolerance=1e-4  nMaxIteration=100  ContinueOnMaxIteration=off  RestoreLinks=warning  ResistiveCurrentMeasurement=off  Frange=[0:2:500]  Ylog=off  Xlog=on  ShowGrid=off  save=off  variable=ZData  structure=VIprim  ZoomFFT=on  StartTime=0.15  cycles=2  DisplayStyle=1  fundamental=50  FreqAxis=on  MaxFrequency=1000  frequencyindicesteady=1  RmsSteady=1  display=off
  prim : spsThreePhaseVIMeasurementLib/Three-Phase V-I Measurement  VoltageMeasurement=phase-to-ground  SetLabelV=on  LabelV=Vprim  Vpu=off  VpuLL=off  CurrentMeasurement=yes  SetLabelI=on  LabelI=Iprim  Ipu=off  Pbase=100e6  Vbase=500e3  OutputType=Complex  PhasorSimulation=off  PSBequivalent=0
  sec : spsThreePhaseVIMeasurementLib/Three-Phase V-I Measurement  VoltageMeasurement=phase-to-ground  SetLabelV=on  LabelV=Vsec  Vpu=off  VpuLL=off  CurrentMeasurement=yes  SetLabelI=on  LabelI=Isec  Ipu=off  Pbase=100e6  Vbase=500e3  OutputType=Complex  PhasorSimulation=off  PSBequivalent=0
  tag scope: IBrk1_EMT=global, IBrk2_EMT=global, Id_ss=global, UBrk1_EMT=global, UBrk2_EMT=global, Uref_ABC=global, Vsrc_ABC=global, m1_dq=global, meas1=global, wt0=global, wt=global
  wires:
  From2/1 -> P (MW)/1
  From4/1 -> Vdc (kV)/1
  From5/1 -> V1 (kV rms LL)/1
  From11/1 -> Q (Mvar)/1
  From/1 -> Uref2m1/1(In1)
  [PQreg_On] -> Control/1(PQreg_ON)
  [Vdc_ref] -> Control/2(Vdc_ref)
  [Qref] -> Control/3(Qref)
  [Vsec] -> Control/4(Vsec)
  [Isec] -> Control/5(Isec)
  Control/1(Uref) -> [Uref_ABC]
  Control/2(Meas) -> [meas1]
  Control/3(m1_dq) -> [m1_dq]
  Control/4(wt) -> [wt]
  [Vsrc_ABC] -> Voltage source/1(In1)
  [wt0] -> DQn->ABC/2(tho)  "theta"
  [VSRC_C] -> DQn->ABC/1(Xdcpnz_c)  "[N+1,18 (6+6+6)]"
  [Vsec] -> Scope8/2
  DQn->ABC/1(Xabc) -> Scope8/1, [Vsrc_ABC]  "Mac_EMT"
  Constant3/1 -> [VSRC_C]
  Gain5/1 -> [wt0]
  Clock/1 -> Gain5/1
  From6/1 -> Voltage source1/1(In1)
  From1/1 -> 3ph SM1/1(Uref_An)
  From7/1 -> 3ph SM1/2(An_Ipos)
  From9/1 -> 3ph SM1/3(An_Icap)
  From27/1 -> Scope2/2  "U_Ap_Dt"
  From28/1 -> Scope2/3  "U_Ap_Dt"
  From102/1 -> Gain4/1  "Ap_Vin"
  From103/1 -> Gain7/1  "Ap_Vbl"
  Status/1 -> Mux9/2  "Status"
  Gain4/1 -> Scope2/4  "Ap_Vin"
  Gain7/1 -> Scope2/5  "Ap_Vbl"
  Mux9/1 -> Scope2/1
  MATLAB Function/2(status) -> Mux9/1
  From44/1 -> MATLAB Function/1(Id)  "U_Ap_Dt"
  From39/1 -> MATLAB Function/2(Vd)  "U_Ap_Dt"
  [Converter2_On] -> Conv 2/1(On)
  ? -> Model2/1(Uswitch)  "USW_Bottom_fcn"
  ? -> Model2/2(status)  "Status_Bottom_Fcn"
  ? -> Model1/1(Uswitch)  "USW_Top"
  ? -> Model1/2(status)  "Status_Top"
  From85/1 -> 3ph SM2/3(Ap_Icap)
  From34/1 -> 3ph SM2/1(Uref_Ap)
  From36/1 -> 3ph SM2/2(Ap_Ipos)
  From91/1 -> Delay10/1  "Ap_Icap"
  From69/1 -> Delay3/1  "U_Ap_SM"
  From90/1 -> Delay11/1  "Ap_Ipos"
  Delay11/1 -> MATLAB Function2/4(Ic)
  Delay10/1 -> MATLAB Function2/3(Ip)
  Delay3/1 -> MATLAB Function2/1(Usm)
  MATLAB Function2/1(UDt) -> Mux24/2  "USW_Top_fcn"
  USW_Top2/1 -> Mux24/1  "USW_Top"
  Mux24/1 -> Scope3/1
  Mux28/1 -> Scope3/2
  USW_Bottom/1 -> Mux28/1  "USW_Bottom"
  MATLAB Function2/3(UDb) -> Mux28/2  "USW_Bottom_fcn"
  Mux29/1 -> Scope3/3
  Status_Top/1 -> Mux29/1  "Status_Top"
  MATLAB Function2/2(Stt) -> Mux29/2  "Status_Top"
  Mux30/1 -> Scope3/4, Scope7/1
  Status_Bottom/1 -> Mux30/1  "Status_Bottom"
  MATLAB Function2/4(Stb) -> Mux30/2  "Status_Bottom_Fcn"
  Mux35/1 -> Scope5/4
  Mux33/1 -> Scope5/2
  Mux34/1 -> Scope5/3
  Mux32/1 -> Scope5/1
  From118/1 -> Mux35/2
  MATLAB Function2/6(IDb) -> Mux33/2  "Db_fcn"
  MATLAB Function2/5(IDt) -> Mux32/2  "Dt_fcn"
  From48/1 -> Mux32/1  "I_Ap_Dt"
  From107/1 -> Mux33/1  "I_Ap_Db"
  USW_Top3/1 -> Mux34/1  "USW_Top"
  Gain1/1 -> Mux34/2
  USW_Bottom1/1 -> Gain1/1  "USW_Bottom"
  From113/1 -> Mux35/1  "I_Ap_Dt"
  From119/1 -> Delay8/1(In1)  "Ap_Ipos"
  Delay9/1(Out1) -> Mux29/3, Subtract/1  "Ipos"
  From120/1 -> Delay9/1(In1)  "Ap_Icap"
  Delay8/1(Out1) -> Gain2/1  "Icap"
  Gain2/1 -> Mux29/4, Subtract/2
  Subtract/1 -> Mux29/5  "Ib"
  From96/1 -> MATLAB Function2/2(Uref)
  MATLAB Function1/1(y) -> Demux6/1, Demux7/1
  Mux23/1 -> MATLAB Function1/1(u), DSS1/1(U)
  Multimeter/1 -> Demux/1
  Demux/2 -> [IBrk2_EMT]
  Demux/1 -> [IBrk1_EMT]
  Demux1/1 -> Mux23/1
  Demux1/2 -> Mux23/2
  Demux1/3 -> Mux23/3
  From8/1 -> Demux1/1
  Demux2/2 -> Mux23/5
  Demux2/3 -> Mux23/6
  Demux2/1 -> Mux23/4
  [V12_Ap] -> Mux23/8
  [V12_Am] -> Mux23/7
  [V12_Bp] -> Mux23/10
  [V12_Bm] -> Mux23/9
  [V12_Cp] -> Mux23/12
  [V12_Cm] -> Mux23/11
  [Vdc2t] -> Mux23/14
  [Vdc2b] -> Mux23/13
  [Vsrc_ABC] -> Demux3/1
  Demux3/1 -> Mux23/15
  Demux3/2 -> Mux23/16
  Demux3/3 -> Mux23/17
  Demux6/3 -> Mux/3
  Demux6/2 -> Mux/2
  Demux6/1 -> Mux/1
  Mux/1 -> Mux12/2, [UBrk1_ss]
  Demux6/6 -> Mux1/3
  Demux6/4 -> Mux1/1
  Mux1/1 -> Mux14/2, [UBrk2_ss]
  Demux6/5 -> Mux1/2
  Mux4/1 -> [Iprim_ss]
  Mux5/1 -> [Isec_ss]
  Mux39/1 -> Rate Transition2/1
  [Vsec] -> Mux39/1  "Vsec_EMT"
  Rate Transition5/1 -> COMPARE1/6
  Rate Transition4/1 -> COMPARE1/5
  Rate Transition3/1 -> COMPARE1/4
  Rate Transition2/1 -> COMPARE1/3
  Rate Transition/1 -> COMPARE1/1
  [Vsec_ss] -> Mux39/2  "Vsec_ss"
  Gain6/1 -> Mux38/2  "Idc_ss"
  [Vdc_ss] -> Mux41/2  "Vdc_ss"
  [Uref_ABC] -> Mux43/1
  [Id_ss] -> Mux42/2  "Idiff_ss"
  Add1/1 -> Gain6/1
  Rate Transition1/1 -> COMPARE1/2
  [Isec] -> Mux40/1  "Isec_EMT"
  Mux42/1 -> Rate Transition4/1
  [Id_abc] -> Mux42/1  "Idiff_EMT"
  [Idc1p_ss] -> Add1/1
  [Uref_ABC_ss] -> Mux43/2
  Mux38/1 -> Rate Transition/1
  [Vdc1] -> Mux41/1  "Vdc_EMT"
  Mux40/1 -> Rate Transition3/1
  [Idc1n_ss] -> Add1/2
  [Idc1] -> Mux38/1  "Idc_EMT"
  Mux41/1 -> Rate Transition1/1
  [Isec_ss] -> Mux40/2  "Isec_ss"
  Mux43/1 -> Rate Transition5/1
  Mux6/1 -> [Ip_ss]
  Mux7/1 -> [In_ss]
  Demux6/13 -> [U_Cp_ss]
  Mux2/1 -> [Vprim_ss]
  Demux6/12 -> [U_Cn_ss]
  Demux6/11 -> [U_Bp_ss]
  Demux6/9 -> [U_Ap_ss]
  Demux6/14 -> Mux2/1
  Demux6/15 -> Mux2/2
  Demux6/8 -> [U_An_ss]
  Demux6/10 -> [U_Bn_ss]
  Demux6/16 -> Mux2/3
  Mux3/1 -> [Vsec_ss]
  Demux6/7 -> [Vdc_ss]
  I->pu1/1 -> [Id_ss]
  [Ip_ss] -> Sum2/1
  Sum2/1 -> I->pu1/1  "Idiff"
  [In_ss] -> Sum2/2
  Demux6/17 -> Mux3/1
  Demux6/18 -> Mux3/2
  Demux6/19 -> Mux3/3
  Demux6/20 -> [Idc1n_ss]
  Demux6/21 -> [Idc1p_ss]
  Demux6/33 -> Mux5/3
  Demux6/32 -> Mux5/2
  Demux6/31 -> Mux5/1
  Demux6/30 -> Mux4/3
  Demux6/29 -> Mux4/2
  Demux6/28 -> Mux4/1
  Demux6/22 -> Mux7/1
  Demux6/24 -> Mux7/2
  Demux6/26 -> Mux7/3
  Demux6/23 -> Mux6/1
  Demux6/25 -> Mux6/2
  Demux6/27 -> Mux6/3
  From10/1 -> Demux2/1
  From26/1 -> Mux13/1  "UBrk1_EMT"
  From33/1 -> Mux13/2  "UBrk2_EMT"
  Multimeter1/1 -> Demux4/1
  Demux4/1 -> Goto13/1, BRK_CTRL/1(UBrk1_EMT)  "UBrk1_EMT"
  From25/1 -> BRK_CTRL/2(Brk_ON)
  From29/1 -> BRK_CTRL1/2(Brk_ON)
  Demux4/2 -> Goto12/1, BRK_CTRL1/1(UBrk1_EMT)  "UBrk2_EMT"
  Mux8/1 -> Scope/1
  Mux10/1 -> Scope/2
  From31/1 -> Mux8/1
  From30/1 -> Mux10/1
  BRK_CTRL/1(IBrk1_ss) -> Mux8/2  "IBrk1_ss"
  BRK_CTRL1/1(IBrk1_ss) -> Mux10/2  "IBrk2_ss"
  [Brk1_On] -> Brk1/1
  [Brk2_On] -> Brk2/1
  [Brk1_On] -> Cast To Double/1
  [Brk2_On] -> Cast To Double1/1
  Mux11/1 -> To Workspace1/1, MATLAB Function1/2(bvec)
  Cast To Double/1 -> Mux11/1
  Cast To Double1/1 -> Mux11/2
  Demux5/2 -> [UBrk2_EMT]
  Demux5/1 -> [UBrk1_EMT]
  Multimeter2/1 -> Demux5/1
  [UBrk1_EMT] -> Mux12/1
  [UBrk2_EMT] -> Mux14/1
  Mux12/1 -> Scope1/1
  Mux14/1 -> Scope1/2
  Demux7/1 -> Demux8/1
  Demux8/1 -> Mux12/3
  Demux8/2 -> Mux14/3
  connections:
  Ld1/LConn1 -- RL Src/RConn1 -- prim/RConn1
  Ld1/LConn2 -- RL Src/RConn2 -- prim/RConn2
  Ld1/LConn3 -- RL Src/RConn3 -- prim/RConn3
  sec/RConn1 -- Ld2/LConn1 -- Tr1/RConn1
  sec/RConn2 -- Ld2/LConn2 -- Tr1/RConn2
  Ld2/LConn3 -- sec/RConn3 -- Tr1/RConn3
  R_startup/RConn1 -- Brk2/RConn1 -- Tr1/LConn1
  R_startup/RConn2 -- Brk2/RConn2 -- Tr1/LConn2
  R_startup/RConn3 -- Brk2/RConn3 -- Tr1/LConn3
  Voltage source/RConn3 -- RL Src/LConn3
  Voltage source/RConn2 -- RL Src/LConn2
  Voltage source/RConn1 -- RL Src/LConn1
  MMC/RConn1 -- MMC_SS/RConn1 -- DC & converter 2/LConn1
  MMC/LConn1 -- MMC_SS/LConn1 -- Voltage source1/RConn1 -- sec/LConn1
  MMC/RConn2 -- MMC_SS/RConn2 -- DC & converter 2/LConn2
  MMC/LConn2 -- MMC_SS/LConn2 -- Voltage source1/RConn2 -- sec/LConn2
  MMC/LConn3 -- MMC_SS/LConn3 -- Voltage source1/RConn3 -- sec/LConn3
  VS Conv2t/LConn1 -- VS Conv2b/RConn1 -- Ground2/LConn1
  Conv 2/LConn1 -- VS Conv2t/RConn1 -- DC & converter 2/RConn1
  Conv 2/LConn2 -- VS Conv2b/LConn1 -- DC & converter 2/RConn2
  Brk1/LConn1 -- prim/LConn1
  Brk1/LConn2 -- prim/LConn2
  Brk1/LConn3 -- prim/LConn3
  R_startup/LConn3 -- Brk2/LConn3 -- Brk1/RConn3
  Brk1/RConn2 -- Brk2/LConn2 -- R_startup/LConn2
  R_startup/LConn1 -- Brk2/LConn1 -- Brk1/RConn1

== system 20240115_HVDCMMCInterconnection/3ph SM1 ==
  Uref_An : Inport
  An_Ipos : Inport  Port=2
  An_Icap : Inport  Port=3
  Demux : Demux  Outputs=2
  Demux2 : Demux  Outputs=2
  Discrete-Time Integrator1 : DiscreteIntegrator  IntegratorMethod=Integration: Trapezoidal  gainval=1  SampleTime=Ts_Power  UpperSaturationLimit=5000  LowerSaturationLimit=500  ICPrevOutput=DiscIntNeverNeededParam  ICPrevScaledInput=DiscIntNeverNeededParam
  Gain1 : Gain  Gain=Nb_PM
  Gain4 : Gain  Gain=1/(C_PM*Nb_PM)
  Gain5 : Gain  Gain=2
  Mux1 : Mux  Inputs=2
  Mux2 : Mux  Inputs=2
  Product3 : Product
  Product4 : Product
  Product7 : Product
  Sum3 : Sum  Inputs=1  InputSameDT=on  SaturateOnIntegerOverflow=on  OutDataTypeStr=Inherit: Same as first input
  Sum4 : Sum  Inputs=+-  InputSameDT=on  SaturateOnIntegerOverflow=on  OutDataTypeStr=Inherit: Same as first input
  Unit Delay5 : UnitDelay  SampleTime=Ts_Power  HasFrameUpgradeWarning=on
  Unit Delay6 : UnitDelay  SampleTime=Ts_Power  HasFrameUpgradeWarning=on
  Unit Delay7 : UnitDelay  SampleTime=Ts_Power  HasFrameUpgradeWarning=on
  An_Vbl : Outport
  An_Vin : Outport  Port=2
  wires:
  Gain5/1 -> Sum4/1
  Gain1/1 -> Demux2/1, Product3/1
  Mux2/1 -> Demux/1
  Demux/1 -> An_Vin/1
  Uref_An/1 -> Gain1/1
  Gain4/1 -> Discrete-Time Integrator1/1
  Mux1/1 -> Unit Delay7/1
  Demux2/2 -> Product7/1
  Unit Delay6/1 -> Gain5/1, Unit Delay5/1
  An_Icap/1 -> Mux1/2
  Demux2/1 -> Product4/1
  Discrete-Time Integrator1/1 -> Unit Delay6/1
  Sum4/1 -> Product7/2, Product4/2  "Vc"
  Unit Delay5/1 -> Sum4/2
  Sum3/1 -> Gain4/1
  Product3/1 -> Sum3/1
  Product4/1 -> Mux2/1  "Vin"
  Demux/2 -> An_Vbl/1
  Product7/1 -> Mux2/2  "Vbl"
  Unit Delay7/1 -> Product3/2
  An_Ipos/1 -> Mux1/1

== system 20240115_HVDCMMCInterconnection/3ph SM2 ==
  Uref_Ap : Inport
  Ap_Ipos : Inport  Port=2
  Ap_Icap : Inport  Port=3
  Demux1 : Demux  Outputs=2
  Demux3 : Demux  Outputs=2
  Discrete-Time Integrator2 : DiscreteIntegrator  IntegratorMethod=Integration: Trapezoidal  gainval=1  SampleTime=Ts_Power  UpperSaturationLimit=5000  LowerSaturationLimit=500  ICPrevOutput=DiscIntNeverNeededParam  ICPrevScaledInput=DiscIntNeverNeededParam
  Gain2 : Gain  Gain=Nb_PM
  Gain3 : Gain  Gain=1/(C_PM*Nb_PM)
  Gain6 : Gain  Gain=2
  Mux3 : Mux  Inputs=2
  Mux4 : Mux  Inputs=2
  Product1 : Product
  Product2 : Product
  Product5 : Product
  Sum1 : Sum  Inputs=1  InputSameDT=on  SaturateOnIntegerOverflow=on  OutDataTypeStr=Inherit: Same as first input
  Sum2 : Sum  Inputs=+-  InputSameDT=on  SaturateOnIntegerOverflow=on  OutDataTypeStr=Inherit: Same as first input
  Unit Delay1 : UnitDelay  SampleTime=Ts_Power  HasFrameUpgradeWarning=on
  Unit Delay2 : UnitDelay  SampleTime=Ts_Power  HasFrameUpgradeWarning=on
  Unit Delay3 : UnitDelay  SampleTime=Ts_Power  HasFrameUpgradeWarning=on
  Ap_Vbl : Outport
  Ap_Vin : Outport  Port=2
  wires:
  Demux1/2 -> Ap_Vbl/1
  Ap_Ipos/1 -> Mux3/1
  Unit Delay3/1 -> Product1/2
  Product1/1 -> Sum1/1
  Sum1/1 -> Gain3/1
  Unit Delay1/1 -> Sum2/2
  Sum2/1 -> Product5/2, Product2/2  "Vc"
  Uref_Ap/1 -> Gain2/1
  Unit Delay2/1 -> Gain6/1, Unit Delay1/1
  Mux3/1 -> Unit Delay3/1
  Demux3/2 -> Product5/1
  Gain3/1 -> Discrete-Time Integrator2/1
  Gain2/1 -> Demux3/1, Product1/1
  Demux3/1 -> Product2/1
  Demux1/1 -> Ap_Vin/1
  Mux4/1 -> Demux1/1
  Product2/1 -> Mux4/1  "Vin"
  Discrete-Time Integrator2/1 -> Unit Delay2/1
  Ap_Icap/1 -> Mux3/2
  Gain6/1 -> Sum2/1
  Product5/1 -> Mux4/2  "Vbl"

== system 20240115_HVDCMMCInterconnection/BRK_CTRL ==
  UBrk1_EMT : Inport
  Brk_ON : Inport  Port=2
  Cast To Double{,1..3} (4 alike) : DataTypeConversion  OutDataTypeStr=double  SaturateOnIntegerOverflow=off  RndMeth=Floor
  Compare To Constant4 : simulink/Logic and Bit Operations/Compare To Constant  relop=>  const=0  OutDataTypeStr=boolean
  Gain : Gain  Gain=1/1e6
  Gain3 : Gain  Gain=1/0.01
  MUX2 : Subsystem
  NOT2 : Logic  Operator=NOT  IconShape=distinctive  AllPortsSameDT=off  OutDataTypeStr=boolean
  Product : Product
  Product1 : Product
  IBrk1_ss : Outport
  wires:
  Cast To Double1/1 -> Product/2
  Product1/1 -> MUX2/2(In2)
  UBrk1_EMT/1 -> Gain3/1, Gain/1
  Compare To Constant4/1 -> Cast To Double1/1, NOT2/1
  Product/1 -> MUX2/1(In1)
  Gain/1 -> Cast To Double3/1
  NOT2/1 -> Cast To Double2/1
  Cast To Double/1 -> Product/1
  Gain3/1 -> Cast To Double/1
  Cast To Double3/1 -> Product1/2
  Brk_ON/1 -> Compare To Constant4/1
  Cast To Double2/1 -> Product1/1
  MUX2/1(Out1) -> IBrk1_ss/1  "IBrk1_ss"

== system 20240115_HVDCMMCInterconnection/BRK_CTRL1 ==
  UBrk1_EMT : Inport
  Brk_ON : Inport  Port=2
  Cast To Double{,1..3} (4 alike) : DataTypeConversion  OutDataTypeStr=double  SaturateOnIntegerOverflow=off  RndMeth=Floor
  Compare To Constant4 : simulink/Logic and Bit Operations/Compare To Constant  relop=>  const=0  OutDataTypeStr=boolean
  Gain : Gain  Gain=1/1e6
  Gain3 : Gain  Gain=1/0.01
  MUX2 : Subsystem
  NOT2 : Logic  Operator=NOT  IconShape=distinctive  AllPortsSameDT=off  OutDataTypeStr=boolean
  Product : Product
  Product1 : Product
  IBrk1_ss : Outport
  wires:
  Cast To Double1/1 -> Product/2
  Product1/1 -> MUX2/2(In2)
  UBrk1_EMT/1 -> Gain3/1, Gain/1
  Compare To Constant4/1 -> Cast To Double1/1, NOT2/1
  Product/1 -> MUX2/1(In1)
  Gain/1 -> Cast To Double3/1
  NOT2/1 -> Cast To Double2/1
  Cast To Double/1 -> Product/1
  Gain3/1 -> Cast To Double/1
  Cast To Double3/1 -> Product1/2
  Brk_ON/1 -> Compare To Constant4/1
  Cast To Double2/1 -> Product1/1
  MUX2/1(Out1) -> IBrk1_ss/1  "IBrk1_ss"
